simulink model "detect_ver1"  (R2016a)
settings: Solver=FixedStepAuto  StartTime=0.0  StopTime=inf  RelTol=1e-3
libraries: embdlinuxlib x2
settings Model: SimulationMode=external  Creator=Yewly  LastModifiedBy=Yewly
settings SolverCC: PositivePriorityOrder=on
settings OptimizationCC: OptimizeModelRefInitCode=on  LifeSpan=Inf  MaxStackSize=64
settings HardwareCC: ProdBitPerPointer=32  ProdLargestAtomicInteger=Long  ProdLargestAtomicFloat=Double  ProdWordSize=32  ProdHWDeviceType=ARM Compatible->ARM Cortex
settings RTWCC: SystemTargetFile=ert.tlc  HardwareBoard=Raspberry Pi  TemplateMakefile=ert_default_tmf  GenerateReport=on  Toolchain=GNU GCC Raspberry Pi  IncludeHyperlinkInReport=on  LaunchReport=on  GenerateTraceInfo=on  GenerateTraceReport=on  GenerateTraceReportSl=on  GenerateTraceReportSf=on  GenerateTraceReportEml=on
settings CodeAppCC: ForceParamTrailComments=on  IgnoreCustomStorageClasses=off  OperatorAnnotations=on  SimulinkDataObjDesc=on  SFDataObjDesc=on  MATLABFcnDesc=on  InsertBlockDesc=on  MATLABSourceComments=on
settings ERTTargetCC: SupportVariableSizeSignals=on

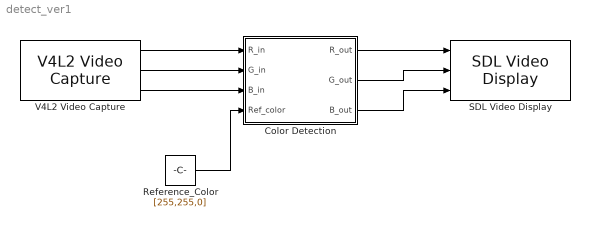
== system detect_ver1 ==
  Color Detection : Subsystem
  Reference_Color : Constant  Value=[255,255,0]  OutDataTypeStr=uint8
  SDL Video Display : embdlinuxlib/SDL Video Display  pixelFormat=RGB  pixelOrder=Planar  rowMajor=on  blockPlatform=Raspberry Pi
  V4L2 Video Capture : embdlinuxlib/V4L2 Video Capture  m_devName='/dev/video0'  roi=[0, 0, 640, 480]  imSizeSelection=640x480  imSize=[640, 480]  pixelFormat=RGB  pixelOrder=Planar  sampleTime=1/30  simOutput=Colorbars  blockPlatform=Raspberry Pi
  wires:
  Reference_Color/1 -> Color Detection/4(Ref_color)
  V4L2 Video Capture/3 -> Color Detection/3(B_in)
  V4L2 Video Capture/2 -> Color Detection/2(G_in)
  V4L2 Video Capture/1 -> Color Detection/1(R_in)
  Color Detection/1(R_out) -> SDL Video Display/1
  Color Detection/2(G_out) -> SDL Video Display/2
  Color Detection/3(B_out) -> SDL Video Display/3

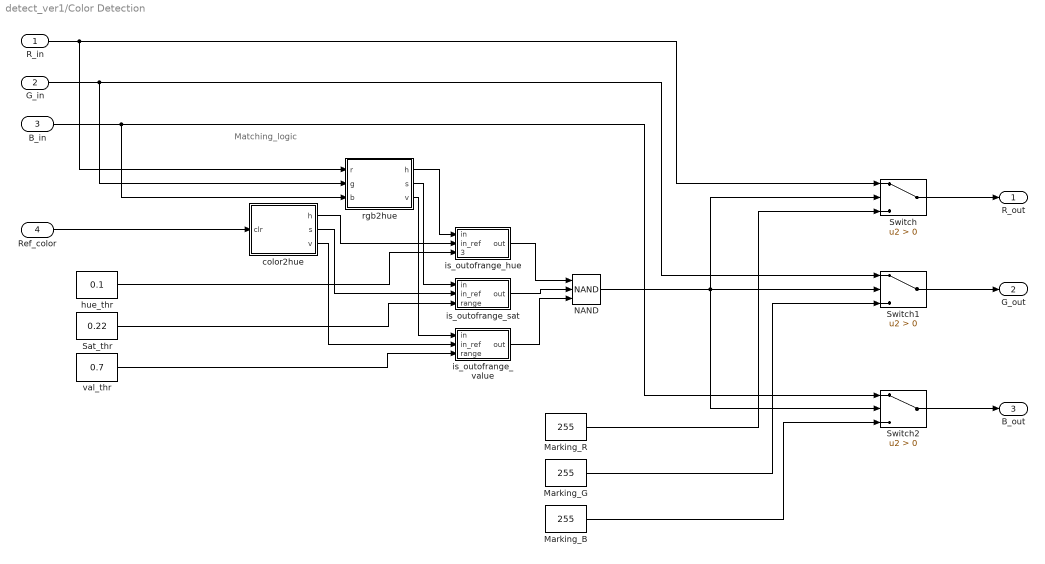
== system detect_ver1/Color Detection ==
  note: Matching_logic
  R_in : Inport
  G_in : Inport  Port=2
  B_in : Inport  Port=3
  Ref_color : Inport  Port=4
  Marking_B : Constant  Value=255
  Marking_G : Constant  Value=255
  Marking_R : Constant  Value=255
  NAND : Logic  Operator=NAND  Inputs=3  IconShape=distinctive  AllPortsSameDT=off  OutDataTypeStr=boolean
  Sat_thr : Constant  Value=0.22
  Switch : Switch  Criteria=u2 > Threshold  OutDataTypeStr=uint8
  Switch1 : Switch  Criteria=u2 > Threshold  OutDataTypeStr=uint8
  Switch2 : Switch  Criteria=u2 > Threshold  OutDataTypeStr=uint8
  color2hue : MATLAB Function  TreatAsAtomicUnit=on
  hue_thr : Constant  Value=0.1
  is_outofrange_hue : Subsystem
  "is_outofrange_sat " : Subsystem
  is_outofrange_value : Subsystem
  rgb2hue : MATLAB Function  TreatAsAtomicUnit=on
  val_thr : Constant  Value=0.7
  R_out : Outport
  G_out : Outport  Port=2
  B_out : Outport  Port=3
  wires:
  NAND/1 -> Switch2/2, Switch1/2, Switch/2
  hue_thr/1 -> is_outofrange_hue/3("threshold ")
  is_outofrange_value/1(out) -> NAND/3
  is_outofrange_hue/1(out) -> NAND/1
  Sat_thr/1 -> "is_outofrange_sat "/3("range ")
  val_thr/1 -> is_outofrange_value/3("range ")
  rgb2hue/3(v) -> is_outofrange_value/1(in)
  color2hue/3(v) -> is_outofrange_value/2(in_ref)
  color2hue/1(h) -> is_outofrange_hue/2(in_ref)
  rgb2hue/1(h) -> is_outofrange_hue/1(in)
  Ref_color/1 -> color2hue/1(clr)
  "is_outofrange_sat "/1(out) -> NAND/2
  color2hue/2(s) -> "is_outofrange_sat "/2(in_ref)
  G_in/1 -> Switch1/1, rgb2hue/2(g)
  rgb2hue/2(s) -> "is_outofrange_sat "/1(in)
  B_in/1 -> Switch2/1, rgb2hue/3(b)
  R_in/1 -> rgb2hue/1(r), Switch/1
  Marking_R/1 -> Switch/3
  Switch/1 -> R_out/1
  Switch1/1 -> G_out/1
  Switch2/1 -> B_out/1
  Marking_G/1 -> Switch1/3
  Marking_B/1 -> Switch2/3

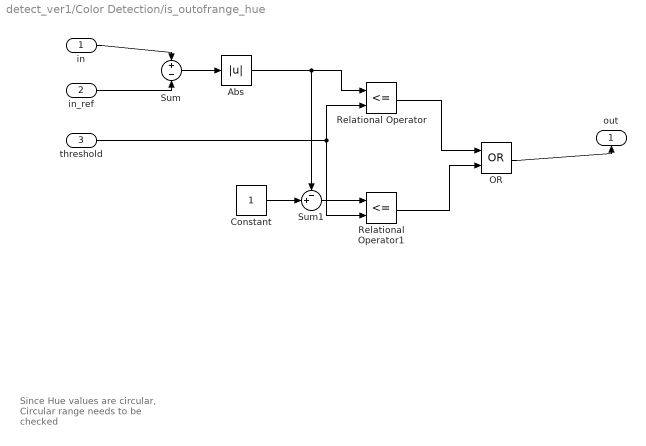
== system detect_ver1/Color Detection/is_outofrange_hue ==
  note: Since Hue values are circular, Circular range needs to be checked
  in : Inport
  in_ref : Inport  Port=2
  "threshold " : Inport  Port=3
  Abs : Abs
  Constant : Constant
  "OR " : Logic  Operator=OR  AllPortsSameDT=off  OutDataTypeStr=boolean
  Relational Operator : RelationalOperator  Operator=<=  OutDataTypeStr=boolean
  Relational Operator1 : RelationalOperator  Operator=<=  OutDataTypeStr=boolean
  Sum : Sum  Inputs=+|-
  Sum1 : Sum  Inputs=-+|
  out : Outport
  wires:
  in/1 -> Sum/1
  in_ref/1 -> Sum/2
  Sum/1 -> Abs/1
  Abs/1 -> Sum1/1, Relational Operator/1
  "threshold "/1 -> Relational Operator1/2, Relational Operator/2
  Constant/1 -> Sum1/2
  Sum1/1 -> Relational Operator1/1
  Relational Operator/1 -> "OR "/1
  Relational Operator1/1 -> "OR "/2
  "OR "/1 -> out/1

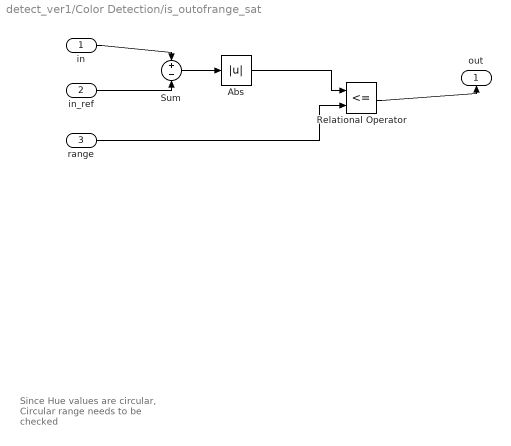
== system detect_ver1/Color Detection/is_outofrange_sat  ==
  note: Since Hue values are circular, Circular range needs to be checked
  in : Inport
  in_ref : Inport  Port=2
  "range " : Inport  Port=3
  Abs : Abs
  Relational Operator : RelationalOperator  Operator=<=  OutDataTypeStr=boolean
  Sum : Sum  Inputs=+|-
  out : Outport
  wires:
  in/1 -> Sum/1
  in_ref/1 -> Sum/2
  Sum/1 -> Abs/1
  Abs/1 -> Relational Operator/1
  "range "/1 -> Relational Operator/2
  Relational Operator/1 -> out/1

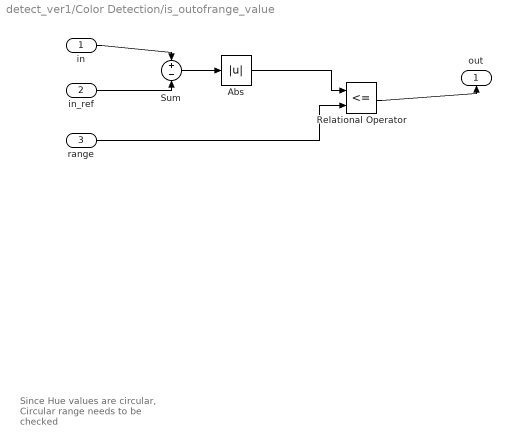
== system detect_ver1/Color Detection/is_outofrange_value ==
  note: Since Hue values are circular, Circular range needs to be checked
  in : Inport
  in_ref : Inport  Port=2
  "range " : Inport  Port=3
  Abs : Abs
  Relational Operator : RelationalOperator  Operator=<=  OutDataTypeStr=boolean
  Sum : Sum  Inputs=+|-
  out : Outport
  wires:
  in/1 -> Sum/1
  in_ref/1 -> Sum/2
  Sum/1 -> Abs/1
  Abs/1 -> Relational Operator/1
  "range "/1 -> Relational Operator/2
  Relational Operator/1 -> out/1

== matlab function detect_ver1/Color Detection/rgb2hue ==
  data: r input; h output; g input; b input; s output; v output
function [h,s,v] = rgb2hue(r,g,b)
%#codegen

sz = size(r);
r_re = double(reshape(r,[sz(1)*sz(2),1]))/255.0;
g_re = double(reshape(g,[sz(1)*sz(2),1]))/255.0;
b_re = double(reshape(b,[sz(1)*sz(2),1]))/255.0;
hsv = rgb2hsv([r_re,g_re,b_re]);
h = reshape(hsv(:,1), sz);
s = reshape(hsv(:,2), sz);
v = reshape(hsv(:,3), sz);

== matlab function detect_ver1/Color Detection/color2hue ==
  data: clr input; h output; s output; v output
function [h,s,v] = color2hue(clr)
%#codegen

hsv = rgb2hsv(double(clr')/255.0);
h = hsv(1);
s = hsv(2);
v = hsv(3);
